simulink model "Mixer"  (R2015a)
settings: Solver=ode2  StartTime=0.0  StopTime=10.0  FixedStep=0.01  RelTol=1e-3
InitFcn:
  | TiltCopter_Parameters_TOSTO_v3
undefined symbols (not defined in the file): b, Kq, Kt, omega_hover
settings Model: Creator=pela  LastModifiedBy=Claudio
settings HardwareCC: ProdLargestAtomicInteger=Long  ProdLargestAtomicFloat=Double  ProdEndianess=LittleEndian  ProdHWDeviceType=ARM Compatible->ARM Cortex
settings RTWCC: GenCodeOnly=on  GenerateReport=on  Toolchain=Microsoft Visual C++ 2013 v12.0 | nmake (64-bit Windows)  BuildConfiguration=Faster Runs  LaunchReport=on  TargetLang=C++
settings GRTTargetCC: MatFileLogging=off  MultiInstanceERTCode=on  CodeInterfacePackaging=C++ class

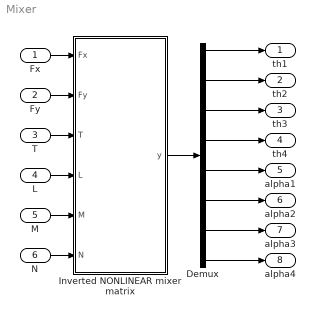
== system Mixer ==
  Fx : Inport
  Fy : Inport  Port=2
  T : Inport  Port=3
  L : Inport  Port=4
  M : Inport  Port=5
  N : Inport  Port=6
  Demux : Demux  Outputs=8
  Inverted NONLINEAR mixer matrix : MATLAB Function  TreatAsAtomicUnit=on
  th1 : Outport
  th2 : Outport  Port=2
  th3 : Outport  Port=3
  "th4 " : Outport  Port=4
  alpha1 : Outport  Port=5
  alpha2 : Outport  Port=6
  alpha3 : Outport  Port=7
  alpha4 : Outport  Port=8
  wires:
  T/1 -> Inverted NONLINEAR mixer matrix/3(T)
  M/1 -> Inverted NONLINEAR mixer matrix/5(M)
  N/1 -> Inverted NONLINEAR mixer matrix/6(N)
  Fx/1 -> Inverted NONLINEAR mixer matrix/1(Fx)
  Fy/1 -> Inverted NONLINEAR mixer matrix/2(Fy)
  L/1 -> Inverted NONLINEAR mixer matrix/4(L)
  Demux/1 -> th1/1
  Demux/2 -> th2/1
  Demux/3 -> th3/1
  Demux/4 -> "th4 "/1
  Demux/5 -> alpha1/1
  Demux/7 -> alpha3/1
  Demux/8 -> alpha4/1
  Demux/6 -> alpha2/1
  Inverted NONLINEAR mixer matrix/1(y) -> Demux/1

== matlab function Mixer/Inverted NONLINEAR mixer matrix ==
  data: Fx input; Fy input; T input; L input; M input; N input; y output; omega_hover parameter; Kt parameter; Kq parameter; b parameter
function y = fcn(Fx,Fy,T,L,M,N,omega_hover,Kt,Kq,b)
%#codegen
alpha_2 = -asin(Fx/(Kt*2*omega_hover^2));

alpha_1 = asin(Fy/(Kt*2*omega_hover^2));
alpha_3 = -alpha_1;
alpha_4 = -alpha_2;

c_alpha1 = cos(alpha_1);
s_alpha1 = sin(alpha_1);
c_alpha2 = cos(alpha_2);
s_alpha2 = sin(alpha_2);
c_alpha3 = cos(alpha_3);
s_alpha3 = sin(alpha_3);
c_alpha4 = cos(alpha_4);
s_alpha4 = sin(alpha_4);


K_inv = [ -(Kq^3*c_alpha2*s_alpha3*s_alpha4 + Kq^3*c_alpha4*s_alpha2*s_alpha3 + Kt^3*b^3*c_alpha2*c_alpha3*s_alpha4 + Kt^3*b^3*c_alpha3*c_alpha4*s_alpha2 - Kq^2*Kt*b*c_alpha2*c_alpha3*s_alpha4 + 2*Kq^2*Kt*b*c_alpha2*c_alpha4*s_alpha3 - Kq^2*Kt*b*c_alpha3*c_alpha4*s_alpha2 - 2*Kq^2*Kt*b*s_alpha2*s_alpha3*s_alpha4 - 2*Kq*Kt^2*b^2*c_alpha2*c_alpha3*c_alpha4 - Kq*Kt^2*b^2*c_alpha2*s_alpha3*s_alpha4 + 2*Kq*Kt^2*b^2*c_alpha3*s_alpha2*s_alpha4 - Kq*Kt^2*b^2*c_alpha4*s_alpha2*s_alpha3)/(2*Kt*(Kq^3*c_alpha1*c_alpha2*s_alpha3*s_alpha4 + Kq^3*c_alpha1*c_alpha4*s_alpha2*s_alpha3 + Kq^3*c_alpha2*c_alpha3*s_alpha1*s_alpha4 + Kq^3*c_alpha3*c_alpha4*s_alpha1*s_alpha2 + Kt^3*b^3*c_alpha1*c_alpha2*c_alpha3*s_alpha4 - Kt^3*b^3*c_alpha1*c_alpha2*c_alpha4*s_alpha3 + Kt^3*b^3*c_alpha1*c_alpha3*c_alpha4*s_alpha2 - Kt^3*b^3*c_alpha2*c_alpha3*c_alpha4*s_alpha1 - 4*Kq*Kt^2*b^2*c_alpha1*c_alpha2*c_alpha3*c_alpha4 - Kq*Kt^2*b^2*c_alpha1*c_alpha2*s_alpha3*s_alpha4 + 2*Kq*Kt^2*b^2*c_alpha1*c_alpha3*s_alpha2*s_alpha4 - Kq*Kt^2*b^2*c_alpha1*c_alpha4*s_alpha2*s_alpha3 - Kq*Kt^2*b^2*c_alpha2*c_alpha3*s_alpha1*s_alpha4 + 2*Kq*Kt^2*b^2*c_alpha2*c_alpha4*s_alpha1*s_alpha3 - Kq*Kt^2*b^2*c_alpha3*c_alpha4*s_alpha1*s_alpha2 - 2*Kq^2*Kt*b*c_alpha1*c_alpha2*c_alpha3*s_alpha4 + 2*Kq^2*Kt*b*c_alpha1*c_alpha2*c_alpha4*s_alpha3 - 2*Kq^2*Kt*b*c_alpha1*c_alpha3*c_alpha4*s_alpha2 + 2*Kq^2*Kt*b*c_alpha2*c_alpha3*c_alpha4*s_alpha1 - Kq^2*Kt*b*c_alpha1*s_alpha2*s_alpha3*s_alpha4 + Kq^2*Kt*b*c_alpha2*s_alpha1*s_alpha3*s_alpha4 - Kq^2*Kt*b*c_alpha3*s_alpha1*s_alpha2*s_alpha4 + Kq^2*Kt*b*c_alpha4*s_alpha1*s_alpha2*s_alpha3)),                                                                                                                                                                                                                                                            (Kt^2*b^2*c_alpha2*c_alpha3*s_alpha4 - Kt^2*b^2*c_alpha3*c_alpha4*s_alpha2 - Kq*Kt*b*c_alpha2*s_alpha3*s_alpha4 + Kq*Kt*b*c_alpha4*s_alpha2*s_alpha3)/(2*(Kq^3*c_alpha1*c_alpha2*s_alpha3*s_alpha4 + Kq^3*c_alpha1*c_alpha4*s_alpha2*s_alpha3 + Kq^3*c_alpha2*c_alpha3*s_alpha1*s_alpha4 + Kq^3*c_alpha3*c_alpha4*s_alpha1*s_alpha2 + Kt^3*b^3*c_alpha1*c_alpha2*c_alpha3*s_alpha4 - Kt^3*b^3*c_alpha1*c_alpha2*c_alpha4*s_alpha3 + Kt^3*b^3*c_alpha1*c_alpha3*c_alpha4*s_alpha2 - Kt^3*b^3*c_alpha2*c_alpha3*c_alpha4*s_alpha1 - 4*Kq*Kt^2*b^2*c_alpha1*c_alpha2*c_alpha3*c_alpha4 - Kq*Kt^2*b^2*c_alpha1*c_alpha2*s_alpha3*s_alpha4 + 2*Kq*Kt^2*b^2*c_alpha1*c_alpha3*s_alpha2*s_alpha4 - Kq*Kt^2*b^2*c_alpha1*c_alpha4*s_alpha2*s_alpha3 - Kq*Kt^2*b^2*c_alpha2*c_alpha3*s_alpha1*s_alpha4 + 2*Kq*Kt^2*b^2*c_alpha2*c_alpha4*s_alpha1*s_alpha3 - Kq*Kt^2*b^2*c_alpha3*c_alpha4*s_alpha1*s_alpha2 - 2*Kq^2*Kt*b*c_alpha1*c_alpha2*c_alpha3*s_alpha4 + 2*Kq^2*Kt*b*c_alpha1*c_alpha2*c_alpha4*s_alpha3 - 2*Kq^2*Kt*b*c_alpha1*c_alpha3*c_alpha4*s_alpha2 + 2*Kq^2*Kt*b*c_alpha2*c_alpha3*c_alpha4*s_alpha1 - Kq^2*Kt*b*c_alpha1*s_alpha2*s_alpha3*s_alpha4 + Kq^2*Kt*b*c_alpha2*s_alpha1*s_alpha3*s_alpha4 - Kq^2*Kt*b*c_alpha3*s_alpha1*s_alpha2*s_alpha4 + Kq^2*Kt*b*c_alpha4*s_alpha1*s_alpha2*s_alpha3)), -(2*Kq^2*c_alpha2*c_alpha3*s_alpha4 + 2*Kq^2*c_alpha3*c_alpha4*s_alpha2 - Kt^2*b^2*c_alpha2*c_alpha3*s_alpha4 + 2*Kt^2*b^2*c_alpha2*c_alpha4*s_alpha3 - Kt^2*b^2*c_alpha3*c_alpha4*s_alpha2 + 4*Kq*Kt*b*c_alpha2*c_alpha3*c_alpha4 + Kq*Kt*b*c_alpha2*s_alpha3*s_alpha4 - 2*Kq*Kt*b*c_alpha3*s_alpha2*s_alpha4 + Kq*Kt*b*c_alpha4*s_alpha2*s_alpha3)/(2*(Kq^3*c_alpha1*c_alpha2*s_alpha3*s_alpha4 + Kq^3*c_alpha1*c_alpha4*s_alpha2*s_alpha3 + Kq^3*c_alpha2*c_alpha3*s_alpha1*s_alpha4 + Kq^3*c_alpha3*c_alpha4*s_alpha1*s_alpha2 + Kt^3*b^3*c_alpha1*c_alpha2*c_alpha3*s_alpha4 - Kt^3*b^3*c_alpha1*c_alpha2*c_alpha4*s_alpha3 + Kt^3*b^3*c_alpha1*c_alpha3*c_alpha4*s_alpha2 - Kt^3*b^3*c_alpha2*c_alpha3*c_alpha4*s_alpha1 - 4*Kq*Kt^2*b^2*c_alpha1*c_alpha2*c_alpha3*c_alpha4 - Kq*Kt^2*b^2*c_alpha1*c_alpha2*s_alpha3*s_alpha4 + 2*Kq*Kt^2*b^2*c_alpha1*c_alpha3*s_alpha2*s_alpha4 - Kq*Kt^2*b^2*c_alpha1*c_alpha4*s_alpha2*s_alpha3 - Kq*Kt^2*b^2*c_alpha2*c_alpha3*s_alpha1*s_alpha4 + 2*Kq*Kt^2*b^2*c_alpha2*c_alpha4*s_alpha1*s_alpha3 - Kq*Kt^2*b^2*c_alpha3*c_alpha4*s_alpha1*s_alpha2 - 2*Kq^2*Kt*b*c_alpha1*c_alpha2*c_alpha3*s_alpha4 + 2*Kq^2*Kt*b*c_alpha1*c_alpha2*c_alpha4*s_alpha3 - 2*Kq^2*Kt*b*c_alpha1*c_alpha3*c_alpha4*s_alpha2 + 2*Kq^2*Kt*b*c_alpha2*c_alpha3*c_alpha4*s_alpha1 - Kq^2*Kt*b*c_alpha1*s_alpha2*s_alpha3*s_alpha4 + Kq^2*Kt*b*c_alpha2*s_alpha1*s_alpha3*s_alpha4 - Kq^2*Kt*b*c_alpha3*s_alpha1*s_alpha2*s_alpha4 + Kq^2*Kt*b*c_alpha4*s_alpha1*s_alpha2*s_alpha3)), (Kq^2*c_alpha2*s_alpha3*s_alpha4 + Kq^2*c_alpha4*s_alpha2*s_alpha3 - 2*Kt^2*b^2*c_alpha2*c_alpha3*c_alpha4 - Kq*Kt*b*c_alpha2*c_alpha3*s_alpha4 + 2*Kq*Kt*b*c_alpha2*c_alpha4*s_alpha3 - Kq*Kt*b*c_alpha3*c_alpha4*s_alpha2)/(2*(Kq^3*c_alpha1*c_alpha2*s_alpha3*s_alpha4 + Kq^3*c_alpha1*c_alpha4*s_alpha2*s_alpha3 + Kq^3*c_alpha2*c_alpha3*s_alpha1*s_alpha4 + Kq^3*c_alpha3*c_alpha4*s_alpha1*s_alpha2 + Kt^3*b^3*c_alpha1*c_alpha2*c_alpha3*s_alpha4 - Kt^3*b^3*c_alpha1*c_alpha2*c_alpha4*s_alpha3 + Kt^3*b^3*c_alpha1*c_alpha3*c_alpha4*s_alpha2 - Kt^3*b^3*c_alpha2*c_alpha3*c_alpha4*s_alpha1 - 4*Kq*Kt^2*b^2*c_alpha1*c_alpha2*c_alpha3*c_alpha4 - Kq*Kt^2*b^2*c_alpha1*c_alpha2*s_alpha3*s_alpha4 + 2*Kq*Kt^2*b^2*c_alpha1*c_alpha3*s_alpha2*s_alpha4 - Kq*Kt^2*b^2*c_alpha1*c_alpha4*s_alpha2*s_alpha3 - Kq*Kt^2*b^2*c_alpha2*c_alpha3*s_alpha1*s_alpha4 + 2*Kq*Kt^2*b^2*c_alpha2*c_alpha4*s_alpha1*s_alpha3 - Kq*Kt^2*b^2*c_alpha3*c_alpha4*s_alpha1*s_alpha2 - 2*Kq^2*Kt*b*c_alpha1*c_alpha2*c_alpha3*s_alpha4 + 2*Kq^2*Kt*b*c_alpha1*c_alpha2*c_alpha4*s_alpha3 - 2*Kq^2*Kt*b*c_alpha1*c_alpha3*c_alpha4*s_alpha2 + 2*Kq^2*Kt*b*c_alpha2*c_alpha3*c_alpha4*s_alpha1 - Kq^2*Kt*b*c_alpha1*s_alpha2*s_alpha3*s_alpha4 + Kq^2*Kt*b*c_alpha2*s_alpha1*s_alpha3*s_alpha4 - Kq^2*Kt*b*c_alpha3*s_alpha1*s_alpha2*s_alpha4 + Kq^2*Kt*b*c_alpha4*s_alpha1*s_alpha2*s_alpha3));
                                                                                                                                                                                                                                                                                                                                                                         -((Kq*s_alpha4 + Kt*b*c_alpha4)*(Kq^2*c_alpha1*s_alpha3 + Kq^2*c_alpha3*s_alpha1 - Kt^2*b^2*c_alpha1*s_alpha3 - Kt^2*b^2*c_alpha3*s_alpha1 + 2*Kq*Kt*b*s_alpha1*s_alpha3 - 2*Kq*Kt*b*c_alpha1*c_alpha3))/(2*Kt*(Kq^3*c_alpha1*c_alpha2*s_alpha3*s_alpha4 + Kq^3*c_alpha1*c_alpha4*s_alpha2*s_alpha3 + Kq^3*c_alpha2*c_alpha3*s_alpha1*s_alpha4 + Kq^3*c_alpha3*c_alpha4*s_alpha1*s_alpha2 + Kt^3*b^3*c_alpha1*c_alpha2*c_alpha3*s_alpha4 - Kt^3*b^3*c_alpha1*c_alpha2*c_alpha4*s_alpha3 + Kt^3*b^3*c_alpha1*c_alpha3*c_alpha4*s_alpha2 - Kt^3*b^3*c_alpha2*c_alpha3*c_alpha4*s_alpha1 - 4*Kq*Kt^2*b^2*c_alpha1*c_alpha2*c_alpha3*c_alpha4 - Kq*Kt^2*b^2*c_alpha1*c_alpha2*s_alpha3*s_alpha4 + 2*Kq*Kt^2*b^2*c_alpha1*c_alpha3*s_alpha2*s_alpha4 - Kq*Kt^2*b^2*c_alpha1*c_alpha4*s_alpha2*s_alpha3 - Kq*Kt^2*b^2*c_alpha2*c_alpha3*s_alpha1*s_alpha4 + 2*Kq*Kt^2*b^2*c_alpha2*c_alpha4*s_alpha1*s_alpha3 - Kq*Kt^2*b^2*c_alpha3*c_alpha4*s_alpha1*s_alpha2 - 2*Kq^2*Kt*b*c_alpha1*c_alpha2*c_alpha3*s_alpha4 + 2*Kq^2*Kt*b*c_alpha1*c_alpha2*c_alpha4*s_alpha3 - 2*Kq^2*Kt*b*c_alpha1*c_alpha3*c_alpha4*s_alpha2 + 2*Kq^2*Kt*b*c_alpha2*c_alpha3*c_alpha4*s_alpha1 - Kq^2*Kt*b*c_alpha1*s_alpha2*s_alpha3*s_alpha4 + Kq^2*Kt*b*c_alpha2*s_alpha1*s_alpha3*s_alpha4 - Kq^2*Kt*b*c_alpha3*s_alpha1*s_alpha2*s_alpha4 + Kq^2*Kt*b*c_alpha4*s_alpha1*s_alpha2*s_alpha3)),  (Kt^2*b^2*c_alpha1*c_alpha4*s_alpha3 - 2*Kq^2*c_alpha3*c_alpha4*s_alpha1 - 2*Kt^2*b^2*c_alpha1*c_alpha3*s_alpha4 - 2*Kq^2*c_alpha1*c_alpha4*s_alpha3 + Kt^2*b^2*c_alpha3*c_alpha4*s_alpha1 + 4*Kq*Kt*b*c_alpha1*c_alpha3*c_alpha4 + Kq*Kt*b*c_alpha1*s_alpha3*s_alpha4 + Kq*Kt*b*c_alpha3*s_alpha1*s_alpha4 - 2*Kq*Kt*b*c_alpha4*s_alpha1*s_alpha3)/(2*(Kq^3*c_alpha1*c_alpha2*s_alpha3*s_alpha4 + Kq^3*c_alpha1*c_alpha4*s_alpha2*s_alpha3 + Kq^3*c_alpha2*c_alpha3*s_alpha1*s_alpha4 + Kq^3*c_alpha3*c_alpha4*s_alpha1*s_alpha2 + Kt^3*b^3*c_alpha1*c_alpha2*c_alpha3*s_alpha4 - Kt^3*b^3*c_alpha1*c_alpha2*c_alpha4*s_alpha3 + Kt^3*b^3*c_alpha1*c_alpha3*c_alpha4*s_alpha2 - Kt^3*b^3*c_alpha2*c_alpha3*c_alpha4*s_alpha1 - 4*Kq*Kt^2*b^2*c_alpha1*c_alpha2*c_alpha3*c_alpha4 - Kq*Kt^2*b^2*c_alpha1*c_alpha2*s_alpha3*s_alpha4 + 2*Kq*Kt^2*b^2*c_alpha1*c_alpha3*s_alpha2*s_alpha4 - Kq*Kt^2*b^2*c_alpha1*c_alpha4*s_alpha2*s_alpha3 - Kq*Kt^2*b^2*c_alpha2*c_alpha3*s_alpha1*s_alpha4 + 2*Kq*Kt^2*b^2*c_alpha2*c_alpha4*s_alpha1*s_alpha3 - Kq*Kt^2*b^2*c_alpha3*c_alpha4*s_alpha1*s_alpha2 - 2*Kq^2*Kt*b*c_alpha1*c_alpha2*c_alpha3*s_alpha4 + 2*Kq^2*Kt*b*c_alpha1*c_alpha2*c_alpha4*s_alpha3 - 2*Kq^2*Kt*b*c_alpha1*c_alpha3*c_alpha4*s_alpha2 + 2*Kq^2*Kt*b*c_alpha2*c_alpha3*c_alpha4*s_alpha1 - Kq^2*Kt*b*c_alpha1*s_alpha2*s_alpha3*s_alpha4 + Kq^2*Kt*b*c_alpha2*s_alpha1*s_alpha3*s_alpha4 - Kq^2*Kt*b*c_alpha3*s_alpha1*s_alpha2*s_alpha4 + Kq^2*Kt*b*c_alpha4*s_alpha1*s_alpha2*s_alpha3)),                                                                                                                                                                                                                                                                                                                                                        ((Kt*b*c_alpha1*s_alpha3 - Kt*b*c_alpha3*s_alpha1)*(Kq*s_alpha4 + Kt*b*c_alpha4))/(2*(Kq^3*c_alpha1*c_alpha2*s_alpha3*s_alpha4 + Kq^3*c_alpha1*c_alpha4*s_alpha2*s_alpha3 + Kq^3*c_alpha2*c_alpha3*s_alpha1*s_alpha4 + Kq^3*c_alpha3*c_alpha4*s_alpha1*s_alpha2 + Kt^3*b^3*c_alpha1*c_alpha2*c_alpha3*s_alpha4 - Kt^3*b^3*c_alpha1*c_alpha2*c_alpha4*s_alpha3 + Kt^3*b^3*c_alpha1*c_alpha3*c_alpha4*s_alpha2 - Kt^3*b^3*c_alpha2*c_alpha3*c_alpha4*s_alpha1 - 4*Kq*Kt^2*b^2*c_alpha1*c_alpha2*c_alpha3*c_alpha4 - Kq*Kt^2*b^2*c_alpha1*c_alpha2*s_alpha3*s_alpha4 + 2*Kq*Kt^2*b^2*c_alpha1*c_alpha3*s_alpha2*s_alpha4 - Kq*Kt^2*b^2*c_alpha1*c_alpha4*s_alpha2*s_alpha3 - Kq*Kt^2*b^2*c_alpha2*c_alpha3*s_alpha1*s_alpha4 + 2*Kq*Kt^2*b^2*c_alpha2*c_alpha4*s_alpha1*s_alpha3 - Kq*Kt^2*b^2*c_alpha3*c_alpha4*s_alpha1*s_alpha2 - 2*Kq^2*Kt*b*c_alpha1*c_alpha2*c_alpha3*s_alpha4 + 2*Kq^2*Kt*b*c_alpha1*c_alpha2*c_alpha4*s_alpha3 - 2*Kq^2*Kt*b*c_alpha1*c_alpha3*c_alpha4*s_alpha2 + 2*Kq^2*Kt*b*c_alpha2*c_alpha3*c_alpha4*s_alpha1 - Kq^2*Kt*b*c_alpha1*s_alpha2*s_alpha3*s_alpha4 + Kq^2*Kt*b*c_alpha2*s_alpha1*s_alpha3*s_alpha4 - Kq^2*Kt*b*c_alpha3*s_alpha1*s_alpha2*s_alpha4 + Kq^2*Kt*b*c_alpha4*s_alpha1*s_alpha2*s_alpha3)),                                                                                                                                                            -((Kq*s_alpha4 + Kt*b*c_alpha4)*(Kq*c_alpha1*s_alpha3 + Kq*c_alpha3*s_alpha1 - 2*Kt*b*c_alpha1*c_alpha3))/(2*(Kq^3*c_alpha1*c_alpha2*s_alpha3*s_alpha4 + Kq^3*c_alpha1*c_alpha4*s_alpha2*s_alpha3 + Kq^3*c_alpha2*c_alpha3*s_alpha1*s_alpha4 + Kq^3*c_alpha3*c_alpha4*s_alpha1*s_alpha2 + Kt^3*b^3*c_alpha1*c_alpha2*c_alpha3*s_alpha4 - Kt^3*b^3*c_alpha1*c_alpha2*c_alpha4*s_alpha3 + Kt^3*b^3*c_alpha1*c_alpha3*c_alpha4*s_alpha2 - Kt^3*b^3*c_alpha2*c_alpha3*c_alpha4*s_alpha1 - 4*Kq*Kt^2*b^2*c_alpha1*c_alpha2*c_alpha3*c_alpha4 - Kq*Kt^2*b^2*c_alpha1*c_alpha2*s_alpha3*s_alpha4 + 2*Kq*Kt^2*b^2*c_alpha1*c_alpha3*s_alpha2*s_alpha4 - Kq*Kt^2*b^2*c_alpha1*c_alpha4*s_alpha2*s_alpha3 - Kq*Kt^2*b^2*c_alpha2*c_alpha3*s_alpha1*s_alpha4 + 2*Kq*Kt^2*b^2*c_alpha2*c_alpha4*s_alpha1*s_alpha3 - Kq*Kt^2*b^2*c_alpha3*c_alpha4*s_alpha1*s_alpha2 - 2*Kq^2*Kt*b*c_alpha1*c_alpha2*c_alpha3*s_alpha4 + 2*Kq^2*Kt*b*c_alpha1*c_alpha2*c_alpha4*s_alpha3 - 2*Kq^2*Kt*b*c_alpha1*c_alpha3*c_alpha4*s_alpha2 + 2*Kq^2*Kt*b*c_alpha2*c_alpha3*c_alpha4*s_alpha1 - Kq^2*Kt*b*c_alpha1*s_alpha2*s_alpha3*s_alpha4 + Kq^2*Kt*b*c_alpha2*s_alpha1*s_alpha3*s_alpha4 - Kq^2*Kt*b*c_alpha3*s_alpha1*s_alpha2*s_alpha4 + Kq^2*Kt*b*c_alpha4*s_alpha1*s_alpha2*s_alpha3));
 -(Kq^3*c_alpha2*s_alpha1*s_alpha4 + Kq^3*c_alpha4*s_alpha1*s_alpha2 + Kt^3*b^3*c_alpha1*c_alpha2*s_alpha4 + Kt^3*b^3*c_alpha1*c_alpha4*s_alpha2 - Kq^2*Kt*b*c_alpha1*c_alpha2*s_alpha4 - Kq^2*Kt*b*c_alpha1*c_alpha4*s_alpha2 + 2*Kq^2*Kt*b*c_alpha2*c_alpha4*s_alpha1 - 2*Kq^2*Kt*b*s_alpha1*s_alpha2*s_alpha4 - 2*Kq*Kt^2*b^2*c_alpha1*c_alpha2*c_alpha4 + 2*Kq*Kt^2*b^2*c_alpha1*s_alpha2*s_alpha4 - Kq*Kt^2*b^2*c_alpha2*s_alpha1*s_alpha4 - Kq*Kt^2*b^2*c_alpha4*s_alpha1*s_alpha2)/(2*Kt*(Kq^3*c_alpha1*c_alpha2*s_alpha3*s_alpha4 + Kq^3*c_alpha1*c_alpha4*s_alpha2*s_alpha3 + Kq^3*c_alpha2*c_alpha3*s_alpha1*s_alpha4 + Kq^3*c_alpha3*c_alpha4*s_alpha1*s_alpha2 + Kt^3*b^3*c_alpha1*c_alpha2*c_alpha3*s_alpha4 - Kt^3*b^3*c_alpha1*c_alpha2*c_alpha4*s_alpha3 + Kt^3*b^3*c_alpha1*c_alpha3*c_alpha4*s_alpha2 - Kt^3*b^3*c_alpha2*c_alpha3*c_alpha4*s_alpha1 - 4*Kq*Kt^2*b^2*c_alpha1*c_alpha2*c_alpha3*c_alpha4 - Kq*Kt^2*b^2*c_alpha1*c_alpha2*s_alpha3*s_alpha4 + 2*Kq*Kt^2*b^2*c_alpha1*c_alpha3*s_alpha2*s_alpha4 - Kq*Kt^2*b^2*c_alpha1*c_alpha4*s_alpha2*s_alpha3 - Kq*Kt^2*b^2*c_alpha2*c_alpha3*s_alpha1*s_alpha4 + 2*Kq*Kt^2*b^2*c_alpha2*c_alpha4*s_alpha1*s_alpha3 - Kq*Kt^2*b^2*c_alpha3*c_alpha4*s_alpha1*s_alpha2 - 2*Kq^2*Kt*b*c_alpha1*c_alpha2*c_alpha3*s_alpha4 + 2*Kq^2*Kt*b*c_alpha1*c_alpha2*c_alpha4*s_alpha3 - 2*Kq^2*Kt*b*c_alpha1*c_alpha3*c_alpha4*s_alpha2 + 2*Kq^2*Kt*b*c_alpha2*c_alpha3*c_alpha4*s_alpha1 - Kq^2*Kt*b*c_alpha1*s_alpha2*s_alpha3*s_alpha4 + Kq^2*Kt*b*c_alpha2*s_alpha1*s_alpha3*s_alpha4 - Kq^2*Kt*b*c_alpha3*s_alpha1*s_alpha2*s_alpha4 + Kq^2*Kt*b*c_alpha4*s_alpha1*s_alpha2*s_alpha3)),                                                                                                                                                                                                                                                            (Kt^2*b^2*c_alpha1*c_alpha2*s_alpha4 - Kt^2*b^2*c_alpha1*c_alpha4*s_alpha2 - Kq*Kt*b*c_alpha2*s_alpha1*s_alpha4 + Kq*Kt*b*c_alpha4*s_alpha1*s_alpha2)/(2*(Kq^3*c_alpha1*c_alpha2*s_alpha3*s_alpha4 + Kq^3*c_alpha1*c_alpha4*s_alpha2*s_alpha3 + Kq^3*c_alpha2*c_alpha3*s_alpha1*s_alpha4 + Kq^3*c_alpha3*c_alpha4*s_alpha1*s_alpha2 + Kt^3*b^3*c_alpha1*c_alpha2*c_alpha3*s_alpha4 - Kt^3*b^3*c_alpha1*c_alpha2*c_alpha4*s_alpha3 + Kt^3*b^3*c_alpha1*c_alpha3*c_alpha4*s_alpha2 - Kt^3*b^3*c_alpha2*c_alpha3*c_alpha4*s_alpha1 - 4*Kq*Kt^2*b^2*c_alpha1*c_alpha2*c_alpha3*c_alpha4 - Kq*Kt^2*b^2*c_alpha1*c_alpha2*s_alpha3*s_alpha4 + 2*Kq*Kt^2*b^2*c_alpha1*c_alpha3*s_alpha2*s_alpha4 - Kq*Kt^2*b^2*c_alpha1*c_alpha4*s_alpha2*s_alpha3 - Kq*Kt^2*b^2*c_alpha2*c_alpha3*s_alpha1*s_alpha4 + 2*Kq*Kt^2*b^2*c_alpha2*c_alpha4*s_alpha1*s_alpha3 - Kq*Kt^2*b^2*c_alpha3*c_alpha4*s_alpha1*s_alpha2 - 2*Kq^2*Kt*b*c_alpha1*c_alpha2*c_alpha3*s_alpha4 + 2*Kq^2*Kt*b*c_alpha1*c_alpha2*c_alpha4*s_alpha3 - 2*Kq^2*Kt*b*c_alpha1*c_alpha3*c_alpha4*s_alpha2 + 2*Kq^2*Kt*b*c_alpha2*c_alpha3*c_alpha4*s_alpha1 - Kq^2*Kt*b*c_alpha1*s_alpha2*s_alpha3*s_alpha4 + Kq^2*Kt*b*c_alpha2*s_alpha1*s_alpha3*s_alpha4 - Kq^2*Kt*b*c_alpha3*s_alpha1*s_alpha2*s_alpha4 + Kq^2*Kt*b*c_alpha4*s_alpha1*s_alpha2*s_alpha3)),  (2*Kq^2*c_alpha1*c_alpha2*s_alpha4 + 2*Kq^2*c_alpha1*c_alpha4*s_alpha2 - Kt^2*b^2*c_alpha1*c_alpha2*s_alpha4 - Kt^2*b^2*c_alpha1*c_alpha4*s_alpha2 + 2*Kt^2*b^2*c_alpha2*c_alpha4*s_alpha1 + 4*Kq*Kt*b*c_alpha1*c_alpha2*c_alpha4 - 2*Kq*Kt*b*c_alpha1*s_alpha2*s_alpha4 + Kq*Kt*b*c_alpha2*s_alpha1*s_alpha4 + Kq*Kt*b*c_alpha4*s_alpha1*s_alpha2)/(2*(Kq^3*c_alpha1*c_alpha2*s_alpha3*s_alpha4 + Kq^3*c_alpha1*c_alpha4*s_alpha2*s_alpha3 + Kq^3*c_alpha2*c_alpha3*s_alpha1*s_alpha4 + Kq^3*c_alpha3*c_alpha4*s_alpha1*s_alpha2 + Kt^3*b^3*c_alpha1*c_alpha2*c_alpha3*s_alpha4 - Kt^3*b^3*c_alpha1*c_alpha2*c_alpha4*s_alpha3 + Kt^3*b^3*c_alpha1*c_alpha3*c_alpha4*s_alpha2 - Kt^3*b^3*c_alpha2*c_alpha3*c_alpha4*s_alpha1 - 4*Kq*Kt^2*b^2*c_alpha1*c_alpha2*c_alpha3*c_alpha4 - Kq*Kt^2*b^2*c_alpha1*c_alpha2*s_alpha3*s_alpha4 + 2*Kq*Kt^2*b^2*c_alpha1*c_alpha3*s_alpha2*s_alpha4 - Kq*Kt^2*b^2*c_alpha1*c_alpha4*s_alpha2*s_alpha3 - Kq*Kt^2*b^2*c_alpha2*c_alpha3*s_alpha1*s_alpha4 + 2*Kq*Kt^2*b^2*c_alpha2*c_alpha4*s_alpha1*s_alpha3 - Kq*Kt^2*b^2*c_alpha3*c_alpha4*s_alpha1*s_alpha2 - 2*Kq^2*Kt*b*c_alpha1*c_alpha2*c_alpha3*s_alpha4 + 2*Kq^2*Kt*b*c_alpha1*c_alpha2*c_alpha4*s_alpha3 - 2*Kq^2*Kt*b*c_alpha1*c_alpha3*c_alpha4*s_alpha2 + 2*Kq^2*Kt*b*c_alpha2*c_alpha3*c_alpha4*s_alpha1 - Kq^2*Kt*b*c_alpha1*s_alpha2*s_alpha3*s_alpha4 + Kq^2*Kt*b*c_alpha2*s_alpha1*s_alpha3*s_alpha4 - Kq^2*Kt*b*c_alpha3*s_alpha1*s_alpha2*s_alpha4 + Kq^2*Kt*b*c_alpha4*s_alpha1*s_alpha2*s_alpha3)), (Kq^2*c_alpha2*s_alpha1*s_alpha4 + Kq^2*c_alpha4*s_alpha1*s_alpha2 - 2*Kt^2*b^2*c_alpha1*c_alpha2*c_alpha4 - Kq*Kt*b*c_alpha1*c_alpha2*s_alpha4 - Kq*Kt*b*c_alpha1*c_alpha4*s_alpha2 + 2*Kq*Kt*b*c_alpha2*c_alpha4*s_alpha1)/(2*(Kq^3*c_alpha1*c_alpha2*s_alpha3*s_alpha4 + Kq^3*c_alpha1*c_alpha4*s_alpha2*s_alpha3 + Kq^3*c_alpha2*c_alpha3*s_alpha1*s_alpha4 + Kq^3*c_alpha3*c_alpha4*s_alpha1*s_alpha2 + Kt^3*b^3*c_alpha1*c_alpha2*c_alpha3*s_alpha4 - Kt^3*b^3*c_alpha1*c_alpha2*c_alpha4*s_alpha3 + Kt^3*b^3*c_alpha1*c_alpha3*c_alpha4*s_alpha2 - Kt^3*b^3*c_alpha2*c_alpha3*c_alpha4*s_alpha1 - 4*Kq*Kt^2*b^2*c_alpha1*c_alpha2*c_alpha3*c_alpha4 - Kq*Kt^2*b^2*c_alpha1*c_alpha2*s_alpha3*s_alpha4 + 2*Kq*Kt^2*b^2*c_alpha1*c_alpha3*s_alpha2*s_alpha4 - Kq*Kt^2*b^2*c_alpha1*c_alpha4*s_alpha2*s_alpha3 - Kq*Kt^2*b^2*c_alpha2*c_alpha3*s_alpha1*s_alpha4 + 2*Kq*Kt^2*b^2*c_alpha2*c_alpha4*s_alpha1*s_alpha3 - Kq*Kt^2*b^2*c_alpha3*c_alpha4*s_alpha1*s_alpha2 - 2*Kq^2*Kt*b*c_alpha1*c_alpha2*c_alpha3*s_alpha4 + 2*Kq^2*Kt*b*c_alpha1*c_alpha2*c_alpha4*s_alpha3 - 2*Kq^2*Kt*b*c_alpha1*c_alpha3*c_alpha4*s_alpha2 + 2*Kq^2*Kt*b*c_alpha2*c_alpha3*c_alpha4*s_alpha1 - Kq^2*Kt*b*c_alpha1*s_alpha2*s_alpha3*s_alpha4 + Kq^2*Kt*b*c_alpha2*s_alpha1*s_alpha3*s_alpha4 - Kq^2*Kt*b*c_alpha3*s_alpha1*s_alpha2*s_alpha4 + Kq^2*Kt*b*c_alpha4*s_alpha1*s_alpha2*s_alpha3));
 -(Kq^3*c_alpha1*s_alpha2*s_alpha3 + Kq^3*c_alpha3*s_alpha1*s_alpha2 - Kt^3*b^3*c_alpha1*c_alpha2*s_alpha3 - Kt^3*b^3*c_alpha2*c_alpha3*s_alpha1 + Kq^2*Kt*b*c_alpha1*c_alpha2*s_alpha3 - 2*Kq^2*Kt*b*c_alpha1*c_alpha3*s_alpha2 + Kq^2*Kt*b*c_alpha2*c_alpha3*s_alpha1 + 2*Kq^2*Kt*b*s_alpha1*s_alpha2*s_alpha3 - 2*Kq*Kt^2*b^2*c_alpha1*c_alpha2*c_alpha3 - Kq*Kt^2*b^2*c_alpha1*s_alpha2*s_alpha3 + 2*Kq*Kt^2*b^2*c_alpha2*s_alpha1*s_alpha3 - Kq*Kt^2*b^2*c_alpha3*s_alpha1*s_alpha2)/(2*Kt*(Kq^3*c_alpha1*c_alpha2*s_alpha3*s_alpha4 + Kq^3*c_alpha1*c_alpha4*s_alpha2*s_alpha3 + Kq^3*c_alpha2*c_alpha3*s_alpha1*s_alpha4 + Kq^3*c_alpha3*c_alpha4*s_alpha1*s_alpha2 + Kt^3*b^3*c_alpha1*c_alpha2*c_alpha3*s_alpha4 - Kt^3*b^3*c_alpha1*c_alpha2*c_alpha4*s_alpha3 + Kt^3*b^3*c_alpha1*c_alpha3*c_alpha4*s_alpha2 - Kt^3*b^3*c_alpha2*c_alpha3*c_alpha4*s_alpha1 - 4*Kq*Kt^2*b^2*c_alpha1*c_alpha2*c_alpha3*c_alpha4 - Kq*Kt^2*b^2*c_alpha1*c_alpha2*s_alpha3*s_alpha4 + 2*Kq*Kt^2*b^2*c_alpha1*c_alpha3*s_alpha2*s_alpha4 - Kq*Kt^2*b^2*c_alpha1*c_alpha4*s_alpha2*s_alpha3 - Kq*Kt^2*b^2*c_alpha2*c_alpha3*s_alpha1*s_alpha4 + 2*Kq*Kt^2*b^2*c_alpha2*c_alpha4*s_alpha1*s_alpha3 - Kq*Kt^2*b^2*c_alpha3*c_alpha4*s_alpha1*s_alpha2 - 2*Kq^2*Kt*b*c_alpha1*c_alpha2*c_alpha3*s_alpha4 + 2*Kq^2*Kt*b*c_alpha1*c_alpha2*c_alpha4*s_alpha3 - 2*Kq^2*Kt*b*c_alpha1*c_alpha3*c_alpha4*s_alpha2 + 2*Kq^2*Kt*b*c_alpha2*c_alpha3*c_alpha4*s_alpha1 - Kq^2*Kt*b*c_alpha1*s_alpha2*s_alpha3*s_alpha4 + Kq^2*Kt*b*c_alpha2*s_alpha1*s_alpha3*s_alpha4 - Kq^2*Kt*b*c_alpha3*s_alpha1*s_alpha2*s_alpha4 + Kq^2*Kt*b*c_alpha4*s_alpha1*s_alpha2*s_alpha3)), -(Kt^2*b^2*c_alpha1*c_alpha2*s_alpha3 - 2*Kq^2*c_alpha2*c_alpha3*s_alpha1 - 2*Kq^2*c_alpha1*c_alpha2*s_alpha3 - 2*Kt^2*b^2*c_alpha1*c_alpha3*s_alpha2 + Kt^2*b^2*c_alpha2*c_alpha3*s_alpha1 + 4*Kq*Kt*b*c_alpha1*c_alpha2*c_alpha3 + Kq*Kt*b*c_alpha1*s_alpha2*s_alpha3 - 2*Kq*Kt*b*c_alpha2*s_alpha1*s_alpha3 + Kq*Kt*b*c_alpha3*s_alpha1*s_alpha2)/(2*(Kq^3*c_alpha1*c_alpha2*s_alpha3*s_alpha4 + Kq^3*c_alpha1*c_alpha4*s_alpha2*s_alpha3 + Kq^3*c_alpha2*c_alpha3*s_alpha1*s_alpha4 + Kq^3*c_alpha3*c_alpha4*s_alpha1*s_alpha2 + Kt^3*b^3*c_alpha1*c_alpha2*c_alpha3*s_alpha4 - Kt^3*b^3*c_alpha1*c_alpha2*c_alpha4*s_alpha3 + Kt^3*b^3*c_alpha1*c_alpha3*c_alpha4*s_alpha2 - Kt^3*b^3*c_alpha2*c_alpha3*c_alpha4*s_alpha1 - 4*Kq*Kt^2*b^2*c_alpha1*c_alpha2*c_alpha3*c_alpha4 - Kq*Kt^2*b^2*c_alpha1*c_alpha2*s_alpha3*s_alpha4 + 2*Kq*Kt^2*b^2*c_alpha1*c_alpha3*s_alpha2*s_alpha4 - Kq*Kt^2*b^2*c_alpha1*c_alpha4*s_alpha2*s_alpha3 - Kq*Kt^2*b^2*c_alpha2*c_alpha3*s_alpha1*s_alpha4 + 2*Kq*Kt^2*b^2*c_alpha2*c_alpha4*s_alpha1*s_alpha3 - Kq*Kt^2*b^2*c_alpha3*c_alpha4*s_alpha1*s_alpha2 - 2*Kq^2*Kt*b*c_alpha1*c_alpha2*c_alpha3*s_alpha4 + 2*Kq^2*Kt*b*c_alpha1*c_alpha2*c_alpha4*s_alpha3 - 2*Kq^2*Kt*b*c_alpha1*c_alpha3*c_alpha4*s_alpha2 + 2*Kq^2*Kt*b*c_alpha2*c_alpha3*c_alpha4*s_alpha1 - Kq^2*Kt*b*c_alpha1*s_alpha2*s_alpha3*s_alpha4 + Kq^2*Kt*b*c_alpha2*s_alpha1*s_alpha3*s_alpha4 - Kq^2*Kt*b*c_alpha3*s_alpha1*s_alpha2*s_alpha4 + Kq^2*Kt*b*c_alpha4*s_alpha1*s_alpha2*s_alpha3)),                                                                                                                                                                                                                                                                                                                                                        ((Kt*b*c_alpha1*s_alpha3 - Kt*b*c_alpha3*s_alpha1)*(Kq*s_alpha2 + Kt*b*c_alpha2))/(2*(Kq^3*c_alpha1*c_alpha2*s_alpha3*s_alpha4 + Kq^3*c_alpha1*c_alpha4*s_alpha2*s_alpha3 + Kq^3*c_alpha2*c_alpha3*s_alpha1*s_alpha4 + Kq^3*c_alpha3*c_alpha4*s_alpha1*s_alpha2 + Kt^3*b^3*c_alpha1*c_alpha2*c_alpha3*s_alpha4 - Kt^3*b^3*c_alpha1*c_alpha2*c_alpha4*s_alpha3 + Kt^3*b^3*c_alpha1*c_alpha3*c_alpha4*s_alpha2 - Kt^3*b^3*c_alpha2*c_alpha3*c_alpha4*s_alpha1 - 4*Kq*Kt^2*b^2*c_alpha1*c_alpha2*c_alpha3*c_alpha4 - Kq*Kt^2*b^2*c_alpha1*c_alpha2*s_alpha3*s_alpha4 + 2*Kq*Kt^2*b^2*c_alpha1*c_alpha3*s_alpha2*s_alpha4 - Kq*Kt^2*b^2*c_alpha1*c_alpha4*s_alpha2*s_alpha3 - Kq*Kt^2*b^2*c_alpha2*c_alpha3*s_alpha1*s_alpha4 + 2*Kq*Kt^2*b^2*c_alpha2*c_alpha4*s_alpha1*s_alpha3 - Kq*Kt^2*b^2*c_alpha3*c_alpha4*s_alpha1*s_alpha2 - 2*Kq^2*Kt*b*c_alpha1*c_alpha2*c_alpha3*s_alpha4 + 2*Kq^2*Kt*b*c_alpha1*c_alpha2*c_alpha4*s_alpha3 - 2*Kq^2*Kt*b*c_alpha1*c_alpha3*c_alpha4*s_alpha2 + 2*Kq^2*Kt*b*c_alpha2*c_alpha3*c_alpha4*s_alpha1 - Kq^2*Kt*b*c_alpha1*s_alpha2*s_alpha3*s_alpha4 + Kq^2*Kt*b*c_alpha2*s_alpha1*s_alpha3*s_alpha4 - Kq^2*Kt*b*c_alpha3*s_alpha1*s_alpha2*s_alpha4 + Kq^2*Kt*b*c_alpha4*s_alpha1*s_alpha2*s_alpha3)),                                                                                                                                                            -((Kq*s_alpha2 + Kt*b*c_alpha2)*(Kq*c_alpha1*s_alpha3 + Kq*c_alpha3*s_alpha1 - 2*Kt*b*c_alpha1*c_alpha3))/(2*(Kq^3*c_alpha1*c_alpha2*s_alpha3*s_alpha4 + Kq^3*c_alpha1*c_alpha4*s_alpha2*s_alpha3 + Kq^3*c_alpha2*c_alpha3*s_alpha1*s_alpha4 + Kq^3*c_alpha3*c_alpha4*s_alpha1*s_alpha2 + Kt^3*b^3*c_alpha1*c_alpha2*c_alpha3*s_alpha4 - Kt^3*b^3*c_alpha1*c_alpha2*c_alpha4*s_alpha3 + Kt^3*b^3*c_alpha1*c_alpha3*c_alpha4*s_alpha2 - Kt^3*b^3*c_alpha2*c_alpha3*c_alpha4*s_alpha1 - 4*Kq*Kt^2*b^2*c_alpha1*c_alpha2*c_alpha3*c_alpha4 - Kq*Kt^2*b^2*c_alpha1*c_alpha2*s_alpha3*s_alpha4 + 2*Kq*Kt^2*b^2*c_alpha1*c_alpha3*s_alpha2*s_alpha4 - Kq*Kt^2*b^2*c_alpha1*c_alpha4*s_alpha2*s_alpha3 - Kq*Kt^2*b^2*c_alpha2*c_alpha3*s_alpha1*s_alpha4 + 2*Kq*Kt^2*b^2*c_alpha2*c_alpha4*s_alpha1*s_alpha3 - Kq*Kt^2*b^2*c_alpha3*c_alpha4*s_alpha1*s_alpha2 - 2*Kq^2*Kt*b*c_alpha1*c_alpha2*c_alpha3*s_alpha4 + 2*Kq^2*Kt*b*c_alpha1*c_alpha2*c_alpha4*s_alpha3 - 2*Kq^2*Kt*b*c_alpha1*c_alpha3*c_alpha4*s_alpha2 + 2*Kq^2*Kt*b*c_alpha2*c_alpha3*c_alpha4*s_alpha1 - Kq^2*Kt*b*c_alpha1*s_alpha2*s_alpha3*s_alpha4 + Kq^2*Kt*b*c_alpha2*s_alpha1*s_alpha3*s_alpha4 - Kq^2*Kt*b*c_alpha3*s_alpha1*s_alpha2*s_alpha4 + Kq^2*Kt*b*c_alpha4*s_alpha1*s_alpha2*s_alpha3))]

Omega_result = K_inv*[T;L;M;N];
y = [Omega_result;alpha_1;alpha_2;alpha_3;alpha_4];
